simulink model "RL_Traction_motor"  (R2023a)
settings: Solver=VariableStepAuto  StartTime=0.0  StopTime=0.25  RelTol=1e-3
model workspace (MAT data in the model file):
  Cdc = 0.001
  Jm = 0.1234
  Ki_id = 710.3004
  Ki_iq = 1061.5
  Ki_omega = 500
  Kp_id = 0.8779
  Kp_iq = 1.0744
  Kp_omega = 20
  L0 = 0.00012184
  Ld = 0.00024368
  LdMatrix = [0.000182 0.00018 0.000178 0.000177 0.000176 0.00017475 0.0001735 0.00017247 0.00017132 0.00016571 0.00016537 0.00016571 ... (735 elements, 21x35)]
  Lq = 0.00029758
  LqMatrix = [0.000217 0.000217 0.000217 0.000217 0.000217 0.0002145 0.000212 0.0002115 0.00021022 0.0002079 0.00020461 0.0002079 ... (735 elements, 21x35)]
  PmMatrix = [0.0363 0.0363 0.0363 0.0363 0.0363 0.0363 0.0363 0.0363 0.0363 0.0363 0.0363 0.0363 ... (735 elements, 21x35)]
  Pmax = 35000
  Rs = 0.010087
  Tmax = 200
  Ts = 5e-06
  Tsc = 0.0001
  V1 = 290
  Vnom = 325
  fsw = 10000
  idVec = [-250 -225 -200 -175 -150 -125 -100 -75 -50 -25 0 25 ... (21 elements, 1x21)]
  iqVec = [-425 -400 -375 -350 -325 -300 -275 -250 -225 -200 -175 -150 ... (35 elements, 1x35)]
  p = 8
  psim = 0.044
undefined symbols (not defined in the file or in its folder): ee_sli_rtmsupport, gcbh, idMatrix, Imax, iqMatrix, rpmVec, TqVec, VdcVec
libraries: fl_lib x19, nesl_utility x13, eeGeneralControl x9, slpidlib x7, ee_lib x6, simulink x3, eeTransforms x2, batteryecm_lib x1, eeDqVoltageLimiter x1, eePwmGeneratorTwoLevel x1, eeResolverToDigitalConverter x1
(part 3 of 3)

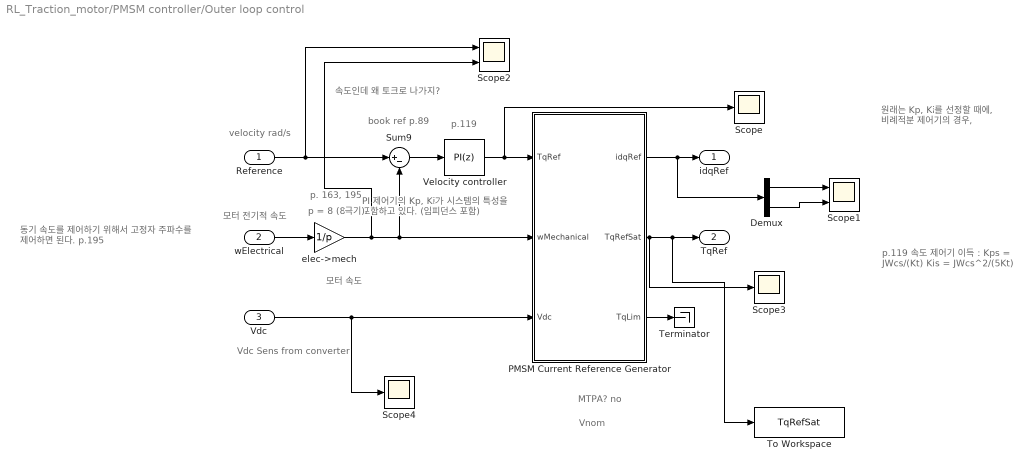
== system RL_Traction_motor/PMSM controller/Outer loop control ==
  note: Vnom
  note: MTPA? no
  note: p.119
      | 속도 제어기 이득 :
      | Kps = JWcs/(Kt)
      | Kis = JWcs^2/(5Kt)
  note: p.119
  note: 원래는 Kp, Ki를 선정할 때에,
      | 비례적분 제어기의 경우,
  note: Vdc Sens
      | from converter
  note: PI 제어기의 Kp, Ki가
      | 시스템의 특성을 포함하고 있다.
      | (임피던스 포함)
  note: 동기 속도를 제어하기 위해서
      | 고정자 주파수를 제어하면 된다. p.195
  note: p. 163, 195
  note: p = 8 (8극기)
  note: 모터 속도
  note: 모터 전기적 속도
  note: velocity rad/s
  note: book ref p.89
  note: 속도인데 왜 토크로 나가지?
  Reference : Inport
  wElectrical : Inport  Port=2
  Vdc : Inport  Port=3
  Demux : Demux  Outputs=2
  PMSM Current Reference Generator : Subsystem  AncestorBlock=eePmsmCurrentReferenceGen/PMSM Current Reference Generator  LoadFcn=ee_sli_rtmsupport( 'loadfcn', gcbh );  mask(PMSM Current Reference Generator){Vnom=Vnom, Pmax=Pmax, Tmax=Tmax, Ts=Tsc, RefType=Zero d-axis control, rpmVec=rpmVec, TqVec=TqVec, VdcVec=VdcVec, PWMMode=SVM: space vector modulation, ModFactor=1, idMatrix=idMatrix, iqMatrix=iqMatrix, p=p, psim=psim, Ld=Ld, Lq=Lq, Rs=Rs, RefExpEnable=0}
      mask prompts: Vnom "physmod:ee:library:comments:control:eePmsmCurrentReferenceGen:NominalDclinkVoltageV_MP"; Pmax "physmod:ee:library:comments:control:eePmsmCurrentReferenceGen:MaximumPowerW_MP"; Tmax "physmod:ee:library:comments:control:eePmsmCurrentReferenceGen:MaximumTorqueNm_MP"; Ts "physmod:ee:library:comments:control:eePmsmCurrentReferenceGen:SampleTime1ForInherited_MP"; RefType "physmod:ee:library:comments:control:eePmsmCurrentReferenceGen:CurrentReferences_MP"; rpmVec "physmod:ee:library:comments:control:eePmsmCurrentReferenceGen:MechanicalSpeedVectorWMechanicalrpm_MP"; TqVec "physmod:ee:library:comments:control:eePmsmCurrentReferenceGen:TorqueReferenceVectorTqRefNm_MP"; VdcVec "physmod:ee:library:comments:control:eePmsmCurrentReferenceGen:DClinkVoltageVectorVdcV_MP"; PWMMode "physmod:ee:library:comments:control:eePmsmCurrentReferenceGen:PWMMethod_MP"; ModFactor "physmod:ee:library:comments:control:eePmsmCurrentReferenceGen:ModulationFactor_MP"; idMatrix "physmod:ee:library:comments:control:eePmsmCurrentReferenceGen:DaxisCurrentReferenceMatrixIdwMechanicalTqRefVdcA_MP"; iqMatrix "physmod:ee:library:comments:control:eePmsmCurrentReferenceGen:QaxisCurrentReferenceMatrixIqwMechanicalTqRefVdcA_MP"; p "physmod:ee:library:comments:control:eePmsmCurrentReferenceGen:NumberOfRotorPolePairs_MP"; psim "physmod:ee:library:comments:control:eePmsmCurrentReferenceGen:PermanentMagnetFluxLinkageWb_MP"; Ld "physmod:ee:library:comments:control:eePmsmCurrentReferenceGen:DaxisInductanceH_MP"; Lq "physmod:ee:library:comments:control:eePmsmCurrentReferenceGen:QaxisInductanceH_MP"; Rs "physmod:ee:library:comments:control:eePmsmCurrentReferenceGen:StatorResistanceOhm_MP"; RefExpEnable "physmod:ee:library:comments:control:eePmsmCurrentReferenceGen:ExportCurrentReferences_MP"
      mask help: physmod:ee:library:comments:control:eePmsmCurrentReferenceGen:PMSMCurrentReferenceGenerator_MD
      mask init:
      | if Vnom <= 0            
      |     error(message('physmod:simscape:compiler:patterns:checks:GreaterThanZero',getString(message('physmod:ee:library:comments:control:eePmsmCurrentReferenceGen:NominalDclinkVoltageV_MP'))));            
      | end
      | if Pmax <= 0            
      |     error(message('physmod:simscape:compiler:patterns:checks:GreaterThanZero',getString(message('physmod:ee:library:comments:control:eePmsmCurrentReferenceGen:MaximumPowerW_MP'))));            
      | end
      | if Tmax <= 0            
      |     error(message('physmod:simscape:compiler:patterns:checks:GreaterThanZero',getString(message('physmod:ee:library:comments:control:eePmsmCurrentReferenceGen:MaximumTorqueNm_MP'))));            
      | end
      | switch RefType
      |     case 'Zero d-axis control'
      |         EnableZDAC = 1;
      |         rpmVec = [0, 3000];
      |         TqVec  = [-100, 0, 100];
      |         VdcVec = [300, 350];
      |         idMatrix = zeros(2,3,2);
      |         iqMatrix = zeros(2,3,2);
      |     case 'Lookup-table based'
      |         EnableZDAC = 0;
      |         if length(rpmVec) < 2            
      |             error(message('physmod:simscape:compiler:patterns:checks:LengthGreaterThanOrEqual',getString(message('physmod:ee:library:comments:control:eePmsmCurrentReferenceGen:MechanicalSpeedVectorWMechanicalrpm_MP')), '2'));            
      |         end
      |         if ~all(diff(rpmVec) > 0)            
      |             error(message('physmod:simscape:compiler:patterns:checks:StrictlyAscendingVec',getString(message('physmod:ee:library:comments:control:eePmsmCurrentReferenceGen:MechanicalSpeedVectorWMechanicalrpm_MP'))));            
      |         end
      |         if length(TqVec) < 2            
      |             error(message('physmod:simscape:compiler:patterns:checks:LengthGreaterThanOrEqual',getString(message('physmod:ee:library:comments:control:eePmsmCurrentReferenceGen:TorqueReferenceVectorTqRefNm_MP')), '2'));            
      |         end
      |         if ~all(diff(TqVec) > 0)            
      |             error(message('physmod:simscape:compiler:patterns:checks:StrictlyAscendingVec',getString(message('physmod:ee:library:comments:control:eePmsmCurrentReferenceGen:TorqueReferenceVectorTqRefNm_MP'))));            
      |         end
      |         if length(VdcVec) < 2            
      |             error(message('physmod:simscape:compiler:patterns:checks:LengthGreaterThanOrEqual',getString(message('physmod:ee:library:comments:control:eePmsmCurrentReferenceGen:DClinkVoltageVectorVdcV_MP')), '2'));            
      |         end
      |         if ~all(diff(VdcVec) > 0)            
      |             error(message('physmod:simscape:compiler:patterns:checks:StrictlyAscendingVec',getString(message('physmod:ee:library:comments:control:eePmsmCurrentReferenceGen:DClinkVoltageVectorVdcV_MP'))));            
      |         end
      |         if ~all(size(idMatrix) == [length(rpmVec), length(TqVec), length(VdcVec)])            
      |             error(message('physmod:simscape:compiler:patterns:checks:Size3DEqual',getString(message('physmod:ee:library:comments:control:eePmsmCurrentReferenceGen:DaxisCurrentReferenceMatrixIdwMechanicalTqRefVdcA_MP')), getString(message('physmod:ee:library:comments:control:eePmsmCurrentReferenceGen:MechanicalSpeedVectorWMechanicalrpm_MP')), getString(message('physmod:ee:library:comments:control:eePmsmCurrentReferenceGen:TorqueReferenceVectorTqRefNm_MP')), getString(message('physmod:ee:library:comments:control:eePmsmCurrentReferenceGen:DClinkVoltageVectorVdcV_MP'))));            
      |         end
      |         if ~all(size(iqMatrix) == [length(rpmVec), length(TqVec), length(VdcVec)])            
      |             error(message('physmod:simscape:compiler:patterns:checks:Size3DEqual',getString(message('physmod:ee:library:comments:control:eePmsmCurrentReferenceGen:QaxisCurrentReferenceMatrixIqwMechanicalTqRefVdcA_MP')), getString(message('physmod:ee:library:comments:control:eePmsmCurrentReferenceGen:MechanicalSpeedVectorWMechanicalrpm_MP')), getString(message('physmod:ee:library:comments:control:eePmsmCurrentReferenceGen:TorqueReferenceVectorTqRefNm_MP')), getString(message('physmod:ee:library:comments:control:eePmsmCurrentReferenceGen:DClinkVoltageVectorVdcV_MP'))));            
      |         end
      |     case 'Automatically generated lookup-table'
      |         EnableZDAC = 0;
      |         if Rs <= 0            
      |             error(message('physmod:simscape:compiler:patterns:checks:GreaterThanZero',getString(message('physmod:ee:library:comments:control:eePmsmCurrentReferenceGen:StatorResistanceOhm_MP'))));            
      |         end
      |         if Ld <= 0            
      |             error(message('physmod:simscape:compiler:patterns:checks:GreaterThanZero',getString(message('physmod:ee:library:comments:control:eePmsmCurrentReferenceGen:DaxisInductanceH_MP'))));            
      |         end
      |         if Lq <= 0            
      |             error(message('physmod:simscape:compiler:patterns:checks:GreaterThanZero',getString(message('physmod:ee:library:comments:control:eePmsmCurrentReferenceGen:QaxisInductanceH_MP'))));            
      |         end
      |         
      |         if ModFactor <= 0            
      |             error(message('physmod:simscape:compiler:patterns:checks:GreaterThanZero',getString(message('physmod:ee:library:comments:control:eePmsmCurrentReferenceGen:ModulationFactor_MP'))));            
      |         end
      |         
      |         if ModFactor > 1            
      |             error(message('physmod:simscape:compiler:patterns:checks:LessThanOrEqual',getString(message('physmod:ee:library:comments:control:eePmsmCurrentReferenceGen:ModulationFactor_MP')),'1'));            
      |         end
      |         
      |         % Check if machine parameters were changed
      |         if exist('pmsm_data', 'var')
      |             dataUpdate = (pmsm_data.Ld   ~= Ld)   ||...
      |                          (pmsm_data.Lq   ~= Lq)   ||...
      |                          (pmsm_data.psim ~= psim) ||...
      |                          (pmsm_data.p    ~= p)    ||...
      |                          (pmsm_data.Rs   ~= Rs)   ||...
      |                          (pmsm_data.Pmax ~= Pmax) ||...
      |                          (pmsm_data.Tmax ~= Tmax) ||...
      |                          (pmsm_data.PWMMode ~= PWMMode) ||...
      |                          (pmsm_data.ModFactor ~= ModFactor);
      |         end
      |         % Check if grid points were changed
      |         if exist('grid_points', 'var')
      |             VecUpdate = max(abs(grid_points.RPM_VECT - rpmVec))~=0 ||...
      |                         max(abs(grid_points.TQ_VECT  - TqVec)) ~=0 ||...
      |                         max(abs(grid_points.VDC_VECT - VdcVec))~=0;
      |         end
      |         % Compute current references only IF current references do not exist OR 
      |         % machine parameters were changed OR grid points were changed
      |         if ~exist('pmsm_ref', 'var') || dataUpdate || VecUpdate
      |             grid_points.RPM_VECT = rpmVec;
      |             grid_points.TQ_VECT  = TqVec;
      |             grid_points.VDC_VECT = VdcVec;
      |             pmsm_data.Ld    = Ld; 
      |             pmsm_data.Lq    = Lq; 
      |             pmsm_data.psim  = psim;   
      |             pmsm_data.p     = p;         
      |             pmsm_data.Rs    = Rs;   
      |             pmsm_data.Pmax  = Pmax;      
      |             pmsm_data.Tbase = Tmax;    
      |             pmsm_data.PWMMode   = PWMMode;      
      |             pmsm_data.ModFactor = ModFactor;
      |             pmsm_ref = ee.control.pmsm.getCurrentReferencesPmsm ( pmsm_data, grid_points );
      |             idMatrix = pmsm_ref.idMatrix;
      |             iqMatrix = pmsm_ref.iqMatrix;
      |         end
      |         % Export current references to base workspace
      |         if RefExpEnable==1
      |             assignin('base', 'pmsm_ref', pmsm_ref)
      |             set_param(gcb,'RefExpEnable','0');
      |         end
      | end
      settings: CopyFcn=ee_sli_rtmsupport( 'copyfcn', gcbh );  DeleteFcn=ee_sli_rtmsupport( 'deletefcn', gcbh );  ModelCloseFcn=ee_sli_rtmsupport( 'modelclosefcn', gcbh );  PostSaveFcn=ee_sli_rtmsupport( 'postsavefcn', gcbh );  PreCopyFcn=ee_sli_rtmsupport( 'precopyfcn', gcbh );  OpenFcn=ee_sli_rtmsupport( 'openfcn', gcbh );  CloseFcn=ee_sli_rtmsupport( 'closefcn', gcbh );  PreDeleteFcn=ee_sli_rtmsupport( 'predeletefcn', gcbh );
      settings: LibrarySourceBlock=|
      | eePmsmCurrentReferenceGen/PMSM Current Reference
      | Generator
      mask Help: web(nesl_help(gcbh))
      mask TypeOptions RefType: physmod:ee:library:comments:control:eePmsmCurrentReferenceGen:ZeroD0x2DAxisControl_PV | physmod:ee:library:comments:control:eePmsmCurrentReferenceGen:Lookup0x2DTableBased_PV | physmod:ee:library:comments:control:eePmsmCurrentReferenceGen:AutomaticallyGeneratedLookup0x2DTable_PV
      mask Callback RefType:
      | % Callback function to set the parameters visibility
      | ee.mask.callbackPopupRefGenPmsm(gcb);
      mask TypeOptions PWMMode: physmod:ee:library:comments:control:eePmsmCurrentReferenceGen:SPWMSinusoidalPWM_PV | physmod:ee:library:comments:control:eePmsmCurrentReferenceGen:SVMSpaceVectorModulation_PV
      mask DialogControl Container2 Prompt: physmod:ee:library:comments:control:eePmsmCurrentReferenceGen:tab_GeneralParameters
      mask DialogControl Vnom Prompt: Nominal dc-link voltage (V)
      mask DialogControl Pmax Prompt: Maximum power (W)
      mask DialogControl Tmax Prompt: Maximum torque (N*m)
      mask DialogControl Ts Prompt: Sample time (-1 for inherited)
      mask DialogControl Container3 Prompt: physmod:ee:library:comments:control:eePmsmCurrentReferenceGen:tab_ReferenceGenStrategy
      mask DialogControl RefType Prompt: Current references
      mask DialogControl rpmVec Prompt: Mechanical speed vector, wMechanical (rpm)
      mask DialogControl TqVec Prompt: Torque reference vector, TqRef (N*m)
      mask DialogControl VdcVec Prompt: DC-link voltage vector, Vdc (V)
      mask DialogControl PWMMode Prompt: PWM method
      mask DialogControl ModFactor Prompt: Modulation factor
      mask DialogControl idMatrix Prompt: D-axis current reference matrix, id(wMechanical,TqRef,Vdc), (A)
      mask DialogControl iqMatrix Prompt: Q-axis current reference matrix, iq(wMechanical,TqRef,Vdc), (A)
      mask DialogControl p Prompt: Number of rotor pole pairs
      mask DialogControl psim Prompt: Permanent magnet flux linkage (Wb)
      mask DialogControl Ld Prompt: D-axis inductance (H)
      mask DialogControl Lq Prompt: Q-axis inductance (H)
      mask DialogControl Rs Prompt: Stator resistance (Ohm)
      mask DialogControl RefExp Prompt: physmod:ee:library:comments:control:eePmsmCurrentReferenceGen:ExportCurrentReferencesToWorkspace_B
      mask DialogControl RefExp Callback:
      | % Enable export of current references
      | set_param(gcb,'RefExpEnable','1');
      mask DialogControl RefExpEnable Prompt: Export current references
  Scope : Scope
  Scope1 : Scope  NumInputPorts=2
  Scope2 : Scope  NumInputPorts=2
  Scope3 : Scope
  Scope4 : Scope
  Sum9 : Sum  Inputs=|+-
  Terminator : Terminator
  To Workspace : ToWorkspace  VariableName=TqRefSat  SampleTime=-1
  Velocity controller : slpidlib/PID Controller  Controller=PI  Form=Parallel  TimeDomain=Discrete-time  UseExternalTs=off  SampleTime=Tsc  IntegratorMethod=Forward Euler  FilterMethod=Forward Euler  ControllerParametersSource=internal  P=Kp_omega  I=Ki_omega  UseKiTs=off  D=0  N=100  UseFilter=on  TunerSelectOption=Transfer Function Based (PID Tuner App)  InitialConditionSource=internal  InitialConditionForIntegrator=0  InitialConditionForFilter=0  DifferentiatorICPrevScaledInput=0  ExternalReset=none  TrackingMode=off  Kt=1  LimitOutput=on  SatLimitsSource=internal  UpperSaturationLimit=Tmax*1.5  LowerSaturationLimit=-Tmax  LinearizeAsGain=on  AntiWindupMode=back-calculation  Kb=1000  LimitIntegrator=off  UpperIntegratorSaturationLimit=inf  LowerIntegratorSaturationLimit=-inf  POutMin=[]  POutMax=[]  IOutMin=[]  IOutMax=[]  DOutMin=[]  DOutMax=[]  NOutMin=[]  NOutMax=[]  SumOutMin=[]  SumOutMax=[]  SaturationOutMin=[]  SaturationOutMax=[]  PParamMin=[]  PParamMax=[]  IParamMin=[]  IParamMax=[]  DParamMin=[]  DParamMax=[]  NParamMin=[]  NParamMax=[]  KbParamMin=[]  KbParamMax=[]  KtParamMin=[]  KtParamMax=[]  KbOutMin=[]  KbOutMax=[]  KtOutMin=[]  KtOutMax=[]  IntegratorOutMin=[]  IntegratorOutMax=[]  FilterOutMin=[]  FilterOutMax=[]  SumI1OutMin=[]  SumI1OutMax=[]  SumI2OutMin=[]  SumI2OutMax=[]  SumI3OutMin=[]  SumI3OutMax=[]  SumI4OutMin=[]  SumI4OutMax=[]  SumDOutMin=[]  SumDOutMax=[]  DifferentiatorOutMin=[]  DifferentiatorOutMax=[]  FilterDiffOutCoefMin=[]  FilterDiffOutCoefMax=[]  ReciprocalOutMin=[]  ReciprocalOutMax=[]  SumDenOutMin=[]  SumDenOutMax=[]  SumNumOutMin=[]  SumNumOutMax=[]  DivideOutMin=[]  DivideOutMax=[]  UdiffTsProdOutMin=[]  UdiffTsProdOutMax=[]  NTsProdOutMin=[]  NTsProdOutMax=[]  UintegralTsProdOutMin=[]  UintegralTsProdOutMax=[]  UngainTsProdOutMin=[]  UngainTsProdOutMax=[]  ClampingZeroOutDataTypeStr=Inherit: Inherit via back propagation  ClampingZeroOutMin=[]  ClampingZeroOutMax=[]  FilterDenConstantOutDataTypeStr=Inherit: Inherit via back propagation  FilterDenConstantOutMin=[]  FilterDenConstantOutMax=[]  PCopyOutDataTypeStr=Inherit: Inherit via back propagation  PCopyOutMin=[]  PCopyOutMax=[]  NCopyOutDataTypeStr=Inherit: Inherit via back propagation  NCopyOutMin=[]  NCopyOutMax=[]  IntegratorContinuousStateAttributes=''  IntegratorStateMustResolveToSignalObject=off  IntegratorRTWStateStorageClass=Auto  FilterContinuousStateAttributes=''  FilterStateMustResolveToSignalObject=off  FilterRTWStateStorageClass=Auto  ParallelPVariant=InternalParameters  IdealPVariant=Disabled  IVariant=InternalParameters  DVariant=Disabled  IntegratorVariant=Discrete  SatVariant=Enabled  AWVariant=BackCalculation  PCopyVariant=Disabled  TRVariant=Disabled  FdbkBlocksVariant=Forward  IdealPFdbkVariant=Disabled  SatFdbkVariant=Disabled  DerivativeFilterVariant=Disabled  NVariant=Disabled  NCopyVariant=Disabled_SignalSpec  FilterICVariant=Disabled  IntegratorICVariant=InternalICs  ExternalResetVariant=Disabled  TRSumVariant=Passthrough  SumFdbkVariant=Disabled  SumVariant=Sum_PI  TsampFilterVariant=InternalTs  TsampNgainVariant=Passthrough  TsampIntegralVariant=Disabled_SignalSpec  ExternalSaturationOutDataTypeStr=Inherit: Same as second input
  elec->mech : Gain  Gain=1/p
  idqRef : Outport  VectorParamsAs1DForOutWhenUnconnected=off
  TqRef : Outport  Port=2  VectorParamsAs1DForOutWhenUnconnected=off
  wires:
  elec->mech/1 -> Scope2/2, Sum9/2, PMSM Current Reference Generator/2(wMechanical)
  PMSM Current Reference Generator/2(TqRefSat) -> To Workspace/1, TqRef/1, Scope3/1
  PMSM Current Reference Generator/1(idqRef) -> Demux/1, idqRef/1
  Vdc/1 -> Scope4/1, PMSM Current Reference Generator/3(Vdc)
  wElectrical/1 -> elec->mech/1
  Reference/1 -> Scope2/1, Sum9/1
  Sum9/1 -> Velocity controller/1
  Velocity controller/1 -> Scope/1, PMSM Current Reference Generator/1(TqRef)
  PMSM Current Reference Generator/3(TqLim) -> Terminator/1
  Demux/1 -> Scope1/1
  Demux/2 -> Scope1/2

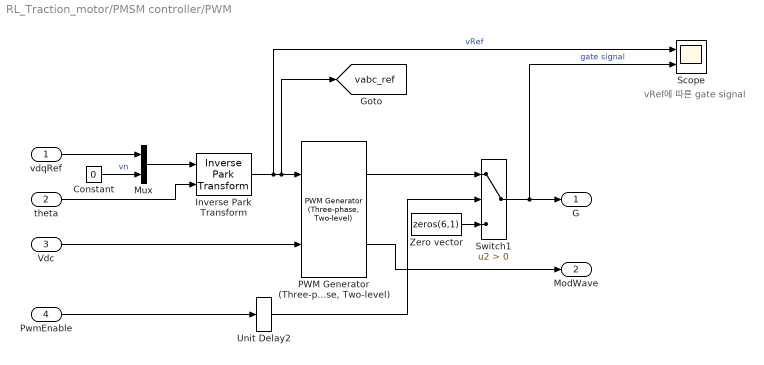
== system RL_Traction_motor/PMSM controller/PWM ==
  note: vRef에 따른 gate signal
  vdqRef : Inport
  theta : Inport  Port=2
  Vdc : Inport  Port=3
  PwmEnable : Inport  Port=4
  Constant : Constant  Value=0  SampleTime=Tsc
  Inverse Park Transform : eeTransforms/Inverse Park Transform  AxisAlignment=Q-axis  PowerInvariant=off
  Mux : Mux  Inputs=2
  "PWM Generator (Three-phase, Two-level)" : eePwmGeneratorTwoLevel/PWM Generator (Three-phase, Two-level)  PWMMode=Continuous PWM (CPWM)  CPWMMode=SVM: space vector modulation  DPWMMode=60 DPWM: 60 degree discontinuous PWM  fsw=fsw  Ts=Ts
  Scope : Scope  NumInputPorts=2
  Switch1 : Switch  Criteria=u2 > Threshold  SaturateOnIntegerOverflow=off  InputSameDT=off
  Unit Delay2 : RateTransition  OutPortSampleTime=5e-06
  Zero vector : Constant  Value=zeros(6,1)  SampleTime=Ts
  G : Outport  VectorParamsAs1DForOutWhenUnconnected=off
  ModWave : Outport  Port=2  SampleTime=Tsc  VectorParamsAs1DForOutWhenUnconnected=off
  tag scope: vabc_ref=global
  wires:
  Unit Delay2/1 -> Switch1/2
  Vdc/1 -> "PWM Generator (Three-phase, Two-level)"/2
  Inverse Park Transform/1 -> Scope/1, [vabc_ref], "PWM Generator (Three-phase, Two-level)"/1  "vRef"
  Switch1/1 -> Scope/2, G/1  "gate signal"
  Zero vector/1 -> Switch1/3
  PwmEnable/1 -> Unit Delay2/1
  "PWM Generator (Three-phase, Two-level)"/1 -> Switch1/1
  "PWM Generator (Three-phase, Two-level)"/2 -> ModWave/1
  Constant/1 -> Mux/2  "vn"
  Mux/1 -> Inverse Park Transform/1
  vdqRef/1 -> Mux/1
  theta/1 -> Inverse Park Transform/2

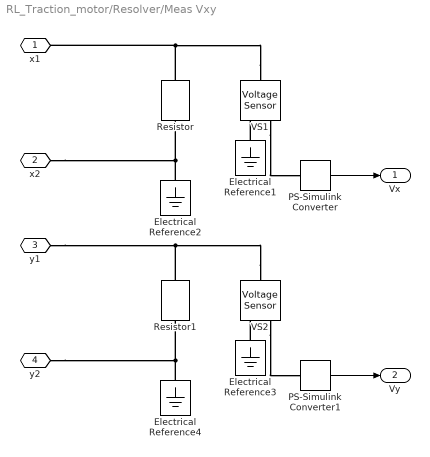
== system RL_Traction_motor/Resolver/Meas Vxy ==
  Electrical Reference{1..4} (4 alike) : fl_lib/Electrical/Electrical Elements/Electrical Reference
  PS-Simulink Converter : nesl_utility/PS-Simulink Converter  PhysicalDomain=network_engine_domain  SubClassName=ps_output  LeftPortType=input  RightPortType=output  PseudoPeriodic=off  Frequencies=[]  VectorFormat=1-D array  Unit=1  AffineConversion=off
  PS-Simulink Converter1 : nesl_utility/PS-Simulink Converter  PhysicalDomain=network_engine_domain  SubClassName=ps_output  LeftPortType=input  RightPortType=output  PseudoPeriodic=off  Frequencies=[]  VectorFormat=1-D array  Unit=1  AffineConversion=off
  Resistor : fl_lib/Electrical/Electrical Elements/Resistor  R=1e3 Ohm  i_specify=off  i_priority=None  i=0 A  i_nominal_specify=off  i_nominal_unit=A  i_nominal_value=1  v_specify=off  v_priority=None  v=0 V  v_nominal_specify=off  v_nominal_unit=V  v_nominal_value=1
  Resistor1 : fl_lib/Electrical/Electrical Elements/Resistor  R=1e3 Ohm  i_specify=off  i_priority=None  i=0 A  i_nominal_specify=off  i_nominal_unit=A  i_nominal_value=1  v_specify=off  v_priority=None  v=0 V  v_nominal_specify=off  v_nominal_unit=V  v_nominal_value=1
  VS1 : fl_lib/Electrical/Electrical Sensors/Voltage Sensor
  VS2 : fl_lib/Electrical/Electrical Sensors/Voltage Sensor
  x1 : PMIOPort  Side=Left
  x2 : PMIOPort  Port=2  Side=Left
  y1 : PMIOPort  Port=3  Side=Left
  y2 : PMIOPort  Port=4  Side=Left
  Vx : Outport  VectorParamsAs1DForOutWhenUnconnected=off
  Vy : Outport  Port=2  VectorParamsAs1DForOutWhenUnconnected=off
  wires:
  PS-Simulink Converter/1 -> Vx/1
  PS-Simulink Converter1/1 -> Vy/1
  connections:
  VS1/LConn1 -- x1/RConn1 -- Resistor/LConn1
  VS1/RConn1 -- PS-Simulink Converter/LConn1
  Resistor/RConn1 -- x2/RConn1 -- Electrical Reference2/LConn1
  Electrical Reference1/LConn1 -- VS1/RConn2
  y2/RConn1 -- Electrical Reference4/LConn1 -- Resistor1/RConn1
  VS2/LConn1 -- y1/RConn1 -- Resistor1/LConn1
  Electrical Reference3/LConn1 -- VS2/RConn2
  VS2/RConn1 -- PS-Simulink Converter1/LConn1

== system RL_Traction_motor/Resolver/Vp ==
  note: Sensor를 작동시키기 위한 voltage Source?
  note: Voltage Sensor
  Electrical Reference1 : fl_lib/Electrical/Electrical Elements/Electrical Reference
  PS-Simulink Converter2 : nesl_utility/PS-Simulink Converter  PhysicalDomain=network_engine_domain  SubClassName=ps_output  LeftPortType=input  RightPortType=output  PseudoPeriodic=off  Frequencies=[]  VectorFormat=1-D array  Unit=1  AffineConversion=off
  VS1 : fl_lib/Electrical/Electrical Sensors/Voltage Sensor
  Vp1 : fl_lib/Electrical/Electrical Sources/AC Voltage Source  amp=5 V  shift=0 rad  frequency=1e4 Hz  omega=0 rad/s
  p1 : PMIOPort  Side=Right
  p2 : PMIOPort  Port=2  Side=Right
  Vp : Outport  VectorParamsAs1DForOutWhenUnconnected=off
  wires:
  PS-Simulink Converter2/1 -> Vp/1
  connections:
  VS1/RConn1 -- PS-Simulink Converter2/LConn1
  Electrical Reference1/LConn1 -- p2/RConn1 -- VS1/RConn2 -- Vp1/RConn1
  VS1/LConn1 -- Vp1/LConn1 -- p1/RConn1

== system RL_Traction_motor/Sensing iabc/Sensor time lag ==
  In1 : Inport
  Demux : Demux  Outputs=3
  Mux : Mux  Inputs=3
  Transfer Fcn : TransferFcn  Denominator=[Ti 1]
  Transfer Fcn1 : TransferFcn  Denominator=[Ti 1]
  Transfer Fcn2 : TransferFcn  Denominator=[Ti 1]
  Out1 : Outport  VectorParamsAs1DForOutWhenUnconnected=off
  wires:
  In1/1 -> Demux/1
  Demux/1 -> Transfer Fcn/1
  Demux/2 -> Transfer Fcn1/1
  Demux/3 -> Transfer Fcn2/1
  Mux/1 -> Out1/1
  Transfer Fcn/1 -> Mux/1
  Transfer Fcn2/1 -> Mux/3
  Transfer Fcn1/1 -> Mux/2

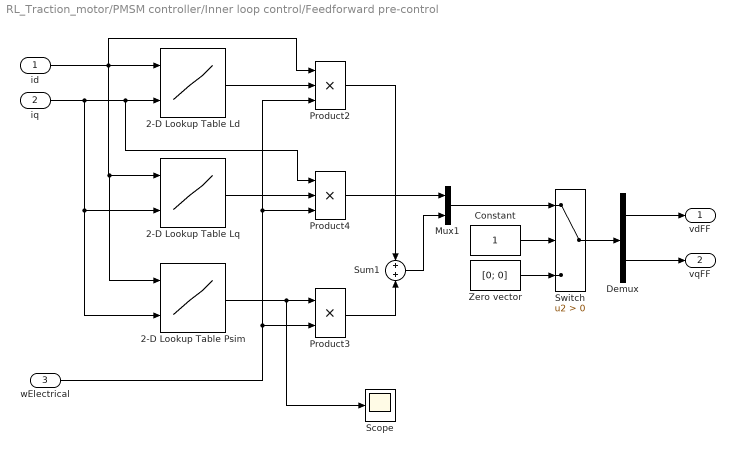
== system RL_Traction_motor/PMSM controller/Inner loop control/Feedforward pre-control ==
  id : Inport
  iq : Inport  Port=2
  wElectrical : Inport  Port=3
  2-D Lookup Table Ld : Lookup_n-D  BreakpointsForDimension1=idVec  BreakpointsForDimension2=iqVec  Table=LdMatrix  ExtrapMethod=Clip  UseLastTableValue=on  InternalRulePriority=Speed  RndMeth=Simplest
      settings: InputPortMap=u0,u1
  2-D Lookup Table Lq : Lookup_n-D  BreakpointsForDimension1=idVec  BreakpointsForDimension2=iqVec  Table=LqMatrix  ExtrapMethod=Clip  InternalRulePriority=Speed  RndMeth=Simplest
      settings: InputPortMap=u0,u1
  2-D Lookup Table Psim : Lookup_n-D  BreakpointsForDimension1=idVec  BreakpointsForDimension2=iqVec  Table=PmMatrix  ExtrapMethod=Clip  InternalRulePriority=Speed  RndMeth=Simplest
      settings: InputPortMap=u0,u1
  Constant : Constant  SampleTime=Tsc
  Demux : Demux  Outputs=2
  Mux1 : Mux  Inputs=2
  Product2 : Product  Inputs=3
  Product3 : Product
  Product4 : Product  Inputs=3
  Scope : Scope
  Sum1 : Sum
  Switch : Switch  Criteria=u2 > Threshold  SaturateOnIntegerOverflow=off  InputSameDT=off
  Zero vector : Constant  Value=[0; 0]  SampleTime=Tsc
  vdFF : Outport  VectorParamsAs1DForOutWhenUnconnected=off
  vqFF : Outport  Port=2  VectorParamsAs1DForOutWhenUnconnected=off
  wires:
  Product3/1 -> Sum1/2
  2-D Lookup Table Lq/1 -> Product4/2
  Constant/1 -> Switch/2
  Switch/1 -> Demux/1
  Demux/1 -> vdFF/1
  Demux/2 -> vqFF/1
  2-D Lookup Table Psim/1 -> Scope/1, Product3/1
  Zero vector/1 -> Switch/3
  Sum1/1 -> Mux1/2
  2-D Lookup Table Ld/1 -> Product2/2
  iq/1 -> Product4/1, 2-D Lookup Table Ld/2, 2-D Lookup Table Lq/2, 2-D Lookup Table Psim/2
  id/1 -> Product2/1, 2-D Lookup Table Psim/1, 2-D Lookup Table Lq/1, 2-D Lookup Table Ld/1
  Product4/1 -> Mux1/1
  Mux1/1 -> Switch/1
  wElectrical/1 -> Product3/2, Product4/3, Product2/3
  Product2/1 -> Sum1/1

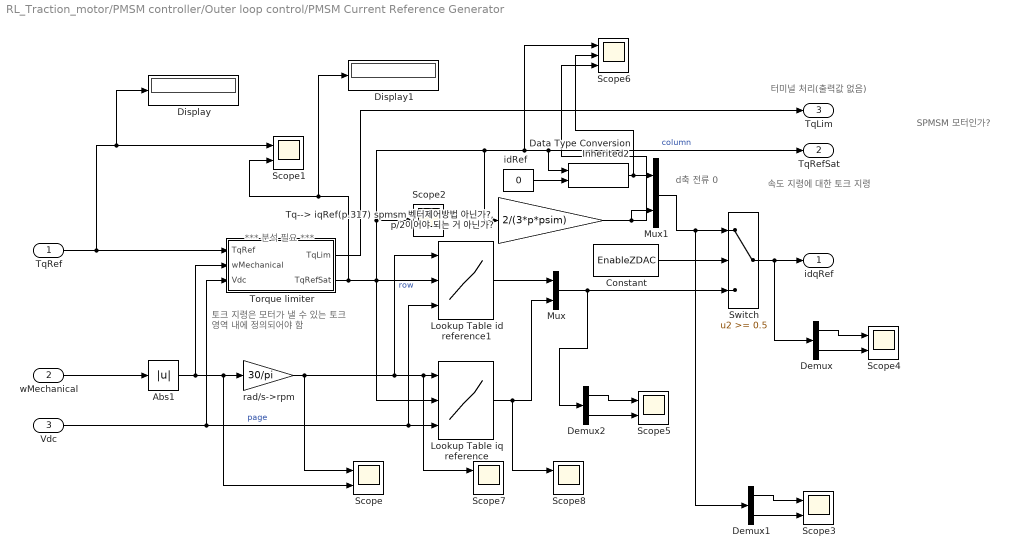
== system RL_Traction_motor/PMSM controller/Outer loop control/PMSM Current Reference Generator ==
  note: SPMSM 모터인가?
  note: d축 전류 0
  note: *** 분석 필요 ***
  note: 토크 지령은 모터가 낼 수 있는
      | 토크 영역 내에 정의되어야 함
  note: 속도 지령에 대한 토크 지령
  note: 터미널 처리(출력값 없음)
  TqRef : Inport  SampleTime=Ts
  wMechanical : Inport  Port=2  SampleTime=Ts
  Vdc : Inport  Port=3  SampleTime=Ts
  Abs1 : Abs  SaturateOnIntegerOverflow=off
  Constant : Constant  Value=EnableZDAC  VectorParams1D=off  SampleTime=Ts
  Data Type Conversion Inherited2 : simulink/Signal Attributes/Data Type Conversion Inherited  ConvertRealWorld=Real World Value  DoSatur=off
  Demux : Demux  Outputs=2
  Demux1 : Demux  Outputs=2
  Demux2 : Demux  Outputs=2
  Display : Display
  Display1 : Display
  Lookup Table id reference1 : Lookup_n-D  NumberOfTableDimensions=3  BreakpointsForDimension1=rpmVec  BreakpointsForDimension2=TqVec  BreakpointsForDimension3=VdcVec  Table=idMatrix
      settings: InputPortMap=u0,u1,u2
  Lookup Table iq reference : Lookup_n-D  NumberOfTableDimensions=3  BreakpointsForDimension1=rpmVec  BreakpointsForDimension2=TqVec  BreakpointsForDimension3=VdcVec  Table=iqMatrix
      settings: InputPortMap=u0,u1,u2
  Mux : Mux  Inputs=2
  Mux1 : Mux  Inputs=2
  Scope{,1,3..5,7..8} (7 alike) : Scope  NumInputPorts=2
  Scope2 : Scope
  Scope6 : Scope  NumInputPorts=3
  Switch : Switch  Threshold=0.5  SaturateOnIntegerOverflow=off  InputSameDT=off
  Torque limiter : Subsystem
  "Tq--> iqRef(p.317) spmsm 벡터제어방법 아닌가?, p/2이어야 되는 거 아닌가? " : Gain  Gain=2/(3*p*psim)
  idRef : Constant  Value=0  SampleTime=Ts
  rad/s->rpm : Gain  Gain=30/pi
  idqRef : Outport  VectorParamsAs1DForOutWhenUnconnected=off
  TqRefSat : Outport  Port=2  VectorParamsAs1DForOutWhenUnconnected=off
  TqLim : Outport  Port=3  VectorParamsAs1DForOutWhenUnconnected=off
  wires:
  idRef/1 -> Data Type Conversion Inherited2/2
  Lookup Table id reference1/1 -> Mux/1
  Lookup Table iq reference/1 -> Scope8/1, Mux/2
  Torque limiter/2(TqRefSat) -> Display1/1, Scope1/2, Lookup Table id reference1/2, Lookup Table iq reference/2, "Tq--> iqRef(p.317) spmsm 벡터제어방법 아닌가?, p/2이어야 되는 거 아닌가? "/1, Scope6/1, TqRefSat/1, Data Type Conversion Inherited2/1, Scope2/1  "column"
  Torque limiter/1(TqLim) -> TqLim/1
  rad/s->rpm/1 -> Scope/1, Lookup Table id reference1/1, Scope7/1, Lookup Table iq reference/1  "row"
  Abs1/1 -> Torque limiter/2(wMechanical), Scope/2, rad/s->rpm/1
  Mux/1 -> Demux2/1, Switch/3
  Switch/1 -> Demux/1, idqRef/1
  Data Type Conversion Inherited2/1 -> Mux1/1, Scope6/2
  "Tq--> iqRef(p.317) spmsm 벡터제어방법 아닌가?, p/2이어야 되는 거 아닌가? "/1 -> Scope6/3, Mux1/2
  TqRef/1 -> Display/1, Scope1/1, Torque limiter/1(TqRef)
  wMechanical/1 -> Abs1/1
  Vdc/1 -> Lookup Table id reference1/3, Lookup Table iq reference/3, Torque limiter/3(Vdc)  "page"
  Constant/1 -> Switch/2
  Demux/2 -> Scope4/2
  Demux/1 -> Scope4/1
  Demux1/2 -> Scope3/2
  Demux1/1 -> Scope3/1
  Mux1/1 -> Demux1/1, Switch/1
  Demux2/2 -> Scope5/2
  Demux2/1 -> Scope5/1

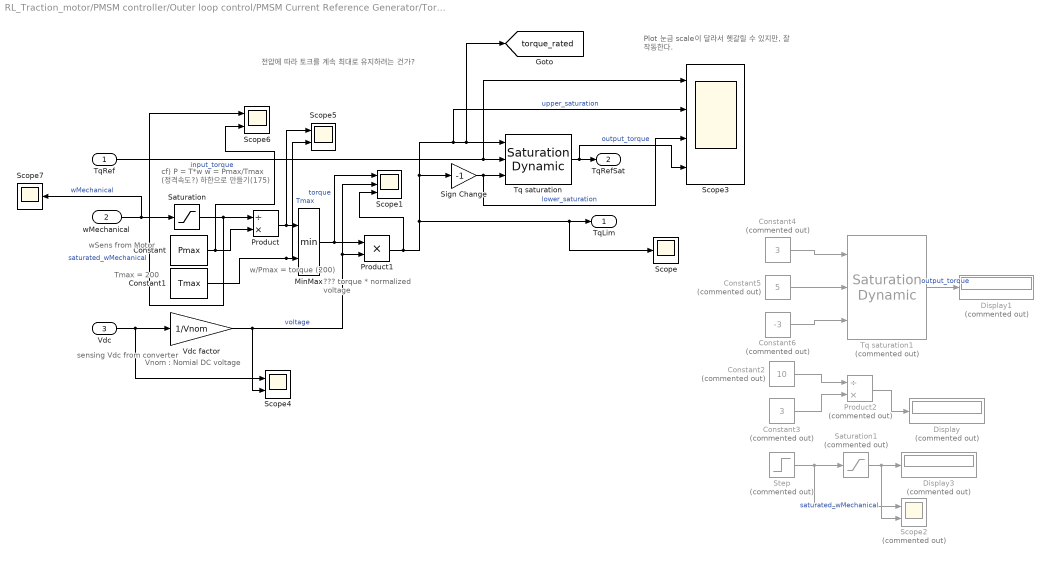
== system RL_Traction_motor/PMSM controller/Outer loop control/PMSM Current Reference Generator/Torque limiter ==
  note: Plot 눈금 scale이 달라서 헷갈릴 수 있지만,
      | 잘 작동한다.
  note: Tmax = 200
  note: 전압에 따라 토크를 계속 최대로 유지하려는 건가?
  note: wSens
      | from Motor
  note: ???
      | torque * normalized voltage
  note: w/Pmax
      | = torque
      | (200)
  note: sensing Vdc
      | from converter
  note: Vnom : Nomial DC voltage
  note: cf) P = T*w
      | w = Pmax/Tmax (정격속도?)
      | 하한으로 만들기(175)
  TqRef : Inport
  wMechanical : Inport  Port=2
  Vdc : Inport  Port=3
  Constant : Constant  Value=Pmax  SampleTime=Ts
  Constant1 : Constant  Value=Tmax  SampleTime=Ts
  Constant2 : Constant  Commented=on  Value=10
  Constant3 : Constant  Commented=on  Value=3
  Constant4 : Constant  Commented=on  Value=3
  Constant5 : Constant  Commented=on  Value=5
  Constant6 : Constant  Commented=on  Value=-3
  Display : Display  Commented=on
  Display1 : Display  Commented=on
  Display3 : Display  Commented=on
  MinMax : MinMax  Inputs=2  OutDataTypeStr=Inherit: Same as first input
  Product : Product  Inputs=/*  OutDataTypeStr=Inherit: Same as first input
  Product1 : Product
  Product2 : Product  Commented=on  Inputs=/*
  Saturation : Saturate  UpperLimit=inf  LowerLimit=Pmax/Tmax
  Saturation1 : Saturate  Commented=on  UpperLimit=inf  LowerLimit=100
  Scope : Scope
  Scope1 : Scope  NumInputPorts=3
  Scope2 : Scope  Commented=on  NumInputPorts=2
  Scope3 : Scope  NumInputPorts=4
  Scope4 : Scope  NumInputPorts=2
  Scope5 : Scope  NumInputPorts=2
  Scope6 : Scope  NumInputPorts=2
  Scope7 : Scope
  Sign Change : Gain  Gain=-1
  Step : Step  Commented=on  Time=0  After=1000  SampleTime=0
  Tq saturation : simulink/Discontinuities/Saturation Dynamic  OutMin=[]  OutMax=[]  OutDataTypeStr=Inherit: Same as second input  OutDataType=fixdt(1, 16)  OutScaling=2^-10  DoSatur=off
  Tq saturation1 : simulink/Discontinuities/Saturation Dynamic  Commented=on  OutMin=[]  OutMax=[]  OutDataTypeStr=Inherit: Same as second input  OutDataType=fixdt(1, 16)  OutScaling=2^-10  DoSatur=off
  Vdc factor : Gain  Gain=1/Vnom
  TqLim : Outport  VectorParamsAs1DForOutWhenUnconnected=off
  TqRefSat : Outport  Port=2  VectorParamsAs1DForOutWhenUnconnected=off
  tag scope: torque_rated=global
  wires:
  Saturation/1 -> Scope6/1, Product/1  "saturated_wMechanical"
  Tq saturation/1 -> Scope3/4, TqRefSat/1  "output_torque"
  Product1/1 -> Scope1/3, Scope3/2, [torque_rated], Tq saturation/1, Sign Change/1, Scope/1, TqLim/1  "upper_saturation"
  TqRef/1 -> Scope3/1, Tq saturation/2  "input_torque"
  Constant1/1 -> Scope5/2, MinMax/2  "Tmax"
  wMechanical/1 -> Scope7/1, Saturation/1  "wMechanical"
  Product/1 -> Scope5/1, MinMax/1
  Sign Change/1 -> Scope3/3, Tq saturation/3  "lower_saturation"
  MinMax/1 -> Scope1/1, Product1/1  "torque"
  Vdc factor/1 -> Scope1/2, Product1/2, Scope4/2  "voltage"
  Constant/1 -> Scope6/2, Product/2
  Step/1 -> Scope2/1, Saturation1/1
  Saturation1/1 -> Scope2/2, Display3/1  "saturated_wMechanical"
  Vdc/1 -> Scope4/1, Vdc factor/1
  Constant2/1 -> Product2/1
  Constant3/1 -> Product2/2
  Product2/1 -> Display/1
  Constant4/1 -> Tq saturation1/1
  Constant5/1 -> Tq saturation1/2
  Constant6/1 -> Tq saturation1/3
  Tq saturation1/1 -> Display1/1  "output_torque"

== matlab function RL_Traction_motor/Subsystem/r(error_norm, constraints) ==
  data: u input; y output
function y = fcn(u)

y = u;

== matlab function RL_Traction_motor/Subsystem/r(error_norm, constraints)1 ==
  data: u input; y output
function y = fcn(u)

y = u;
